simulink model "kadai52"  (R2021b)
settings: Solver=VariableStepAuto  StartTime=0.0  StopTime=40  MaxStep=0.001  RelTol=2.8e-14
settings Model: NumberOfSteps=1000000  Creator=is221042  LastModifiedBy=tomotomo

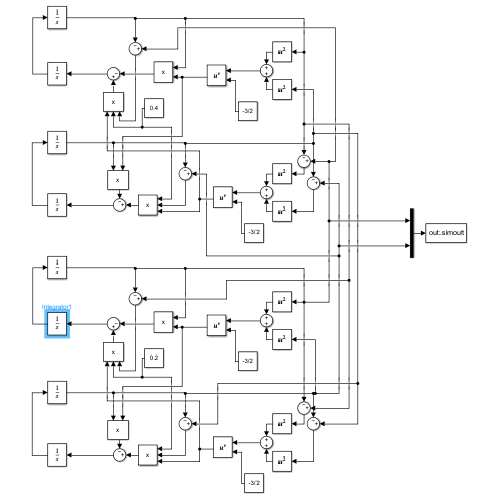
[thumbnail: Simulink's stored preview of the top-level diagram]
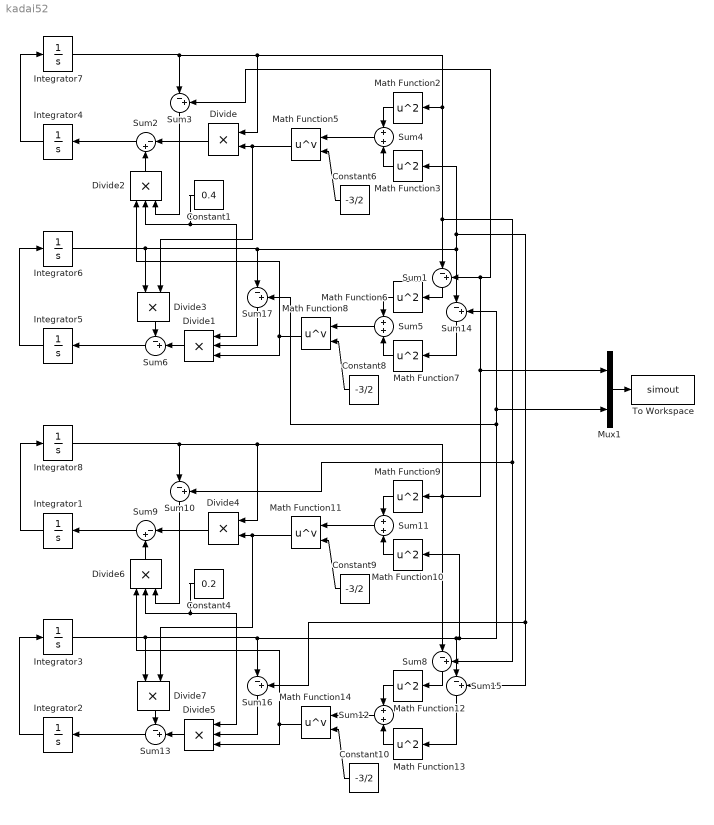
== system kadai52 ==
  Constant1 : Constant  Value=0.4
  Constant{6,8..10} (4 alike) : Constant  Value=-3/2
  Constant4 : Constant  Value=0.2
  Divide{,3..4,7} (4 alike) : Product  Inputs=**
  Divide{1..2,5..6} (4 alike) : Product  Inputs=***
  Integrator1 : Integrator  InitialCondition=0.0
  Integrator2 : Integrator  InitialCondition=1.0
  Integrator3 : Integrator  InitialCondition=0.0
  Integrator4 : Integrator  InitialCondition=2.5
  Integrator5 : Integrator  InitialCondition=1.0
  Integrator6 : Integrator  InitialCondition=0.141421356
  Integrator7 : Integrator  InitialCondition=0.141421356
  Integrator8 : Integrator  InitialCondition=1.0
  Math Function{2..3,6..7,9..10,12..13} (8 alike) : Math  Operator=square  SaturateOnIntegerOverflow=on
  Math Function{5,8,11,14} (4 alike) : Math  Operator=pow  SaturateOnIntegerOverflow=on
  Mux1 : Mux  Inputs=2
  Sum{1..3,8..10,14..17} (10 alike) : Sum  Inputs=|-+
  Sum{4..5,11..12} (4 alike) : Sum  Inputs=+|+
  Sum13 : Sum  Inputs=-+|
  Sum6 : Sum  Inputs=-+|
  To Workspace : ToWorkspace  VariableName=simout  SaveFormat=Timeseries  SampleTime=-1
  wires:
  Divide/1 -> Sum2/1
  Constant1/1 -> Divide1/1, Divide2/2
  Sum3/1 -> Divide2/3
  Divide1/1 -> Sum6/2
  Divide2/1 -> Sum2/2
  Divide3/1 -> Sum6/1
  Sum2/1 -> Integrator4/1
  Sum1/1 -> Math Function6/1
  Integrator5/1 -> Integrator6/1
  Constant8/1 -> Math Function8/2
  Sum4/1 -> Math Function5/1
  Integrator4/1 -> Integrator7/1
  Math Function5/1 -> Divide3/2, Divide/2
  Math Function3/1 -> Sum4/2
  Math Function6/1 -> Sum5/1
  Math Function7/1 -> Sum5/2
  Constant6/1 -> Math Function5/2
  Sum5/1 -> Math Function8/1
  Math Function8/1 -> Divide1/3, Divide2/1
  Math Function2/1 -> Sum4/1
  Integrator8/1 -> Sum10/1, Divide4/1, Sum8/1, Mux1/1, Sum3/2, Sum1/2, Math Function9/1
  Sum6/1 -> Integrator5/1
  Integrator3/1 -> Divide7/1, Sum16/1, Sum15/1, Math Function10/1, Sum14/2, Mux1/2, Sum17/2
  Sum13/1 -> Integrator2/1
  Integrator7/1 -> Sum3/1, Divide/1, Sum1/1, Sum8/2, Sum10/2, Math Function2/1
  Math Function14/1 -> Divide5/3, Divide6/1
  Sum12/1 -> Math Function14/1
  Math Function9/1 -> Sum11/1
  Math Function13/1 -> Sum12/2
  Constant9/1 -> Math Function11/2
  Math Function12/1 -> Sum12/1
  Math Function11/1 -> Divide7/2, Divide4/2
  Math Function10/1 -> Sum11/2
  Sum8/1 -> Math Function12/1
  Divide7/1 -> Sum13/1
  Sum11/1 -> Math Function11/1
  Integrator1/1 -> Integrator8/1
  Sum9/1 -> Integrator1/1
  Integrator2/1 -> Integrator3/1
  Constant10/1 -> Math Function14/2
  Divide6/1 -> Sum9/2
  Divide5/1 -> Sum13/2
  Constant4/1 -> Divide5/1, Divide6/2
  Sum10/1 -> Divide6/3
  Divide4/1 -> Sum9/1
  Sum14/1 -> Math Function7/1
  Sum15/1 -> Math Function13/1
  Integrator6/1 -> Divide3/1, Sum17/1, Sum14/1, Sum15/2, Sum16/2, Math Function3/1
  Sum16/1 -> Divide5/2
  Sum17/1 -> Divide1/2
  Mux1/1 -> To Workspace/1
